simulink model "Continuity"  (R2024b)
settings: Solver=VariableStepAuto  StartTime=0.0  StopTime=10.0  RelTol=1e-3
values from neighbouring files (symbols this model uses):
  A2 = 0.000001    (= 1e-06)    [Continuity_Variable.m]
  p = 1060    [Continuity_Variable.m]
  P1 = 16000    [Continuity_Variable.m]
  Q = 0.0000015    (= 1.5e-06)    [Continuity_Variable.m]
settings Model: Creator=Stephon Woodson  LastModifiedBy=Stephon Woodson

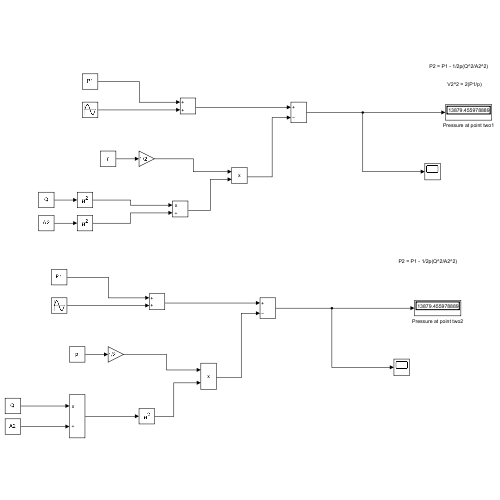
[thumbnail: Simulink's stored preview of the top-level diagram]
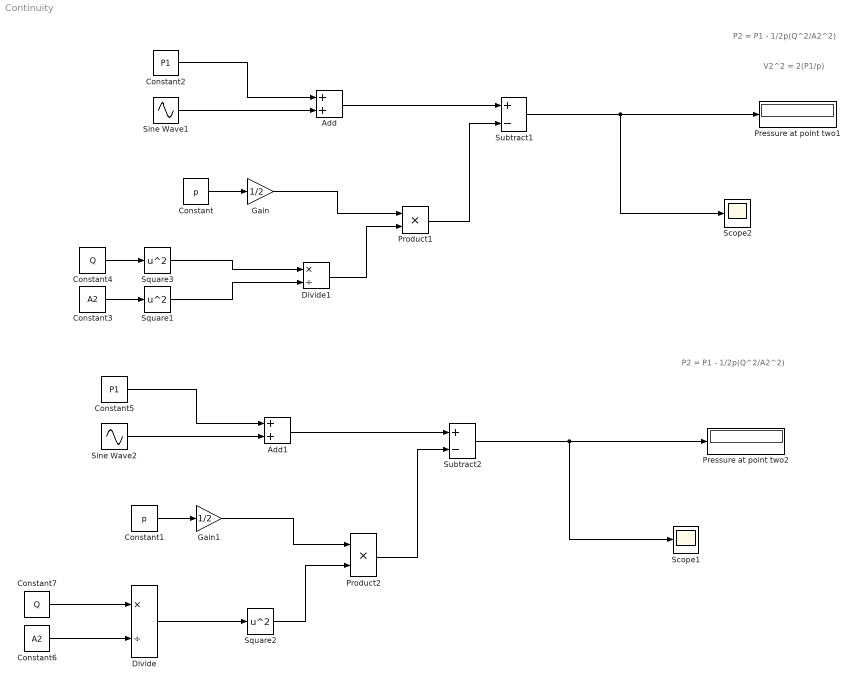
== system Continuity ==
  note: P2 = P1 - 1/2p(Q^2/A2^2)
  note: V2^2 = 2(P1/p)
  note: P2 = P1 - 1/2p(Q^2/A2^2)
  Add : Sum
  Add1 : Sum
  Constant : Constant  Value=p
  Constant1 : Constant  Value=p
  Constant2 : Constant  Value=P1
  Constant3 : Constant  Value=A2
  Constant4 : Constant  Value=Q
  Constant5 : Constant  Value=P1
  Constant6 : Constant  Value=A2
  Constant7 : Constant  Value=Q
  Divide : Product  Inputs=*/
  Divide1 : Product  Inputs=*/
  Gain : Gain  Gain=1/2
  Gain1 : Gain  Gain=1/2
  Pressure at point two1 : Display
  Pressure at point two2 : Display
  Product1 : Product
  Product2 : Product
  Scope1 : Scope
  Scope2 : Scope
  Sine Wave1 : Sin  SampleTime=0
  Sine Wave2 : Sin  SampleTime=0
  Square1 : Math  Operator=square
  Square2 : Math  Operator=square
  Square3 : Math  Operator=square
  Subtract1 : Sum  Inputs=+-
  Subtract2 : Sum  Inputs=+-
  wires:
  Product1/1 -> Subtract1/2
  Subtract1/1 -> Scope2/1, Pressure at point two1/1
  Add/1 -> Subtract1/1
  Constant2/1 -> Add/1
  Constant/1 -> Gain/1
  Gain/1 -> Product1/1
  Sine Wave1/1 -> Add/2
  Constant4/1 -> Square3/1
  Constant3/1 -> Square1/1
  Square1/1 -> Divide1/2
  Square3/1 -> Divide1/1
  Divide1/1 -> Product1/2
  Square2/1 -> Product2/2
  Divide/1 -> Square2/1
  Product2/1 -> Subtract2/2
  Sine Wave2/1 -> Add1/2
  Gain1/1 -> Product2/1
  Constant5/1 -> Add1/1
  Constant1/1 -> Gain1/1
  Subtract2/1 -> Scope1/1, Pressure at point two2/1
  Add1/1 -> Subtract2/1
  Constant6/1 -> Divide/2
  Constant7/1 -> Divide/1
